simulink model "bbbbbbbb"  (R2018b)
settings: Solver=VariableStepAuto  StartTime=0.0  StopTime=20  MaxStep=0.01  RelTol=1e-3
values from neighbouring files (symbols this model uses):
  A = [0 1; 4 0]    [snatch3.m]    (also in snatch4.m; snatch5.m; snatch6.m)
  B = [1; 1]    [snatch3.m]    (also in snatch4.m; snatch5.m; snatch6.m)
  C = [3 0]    [snatch3.m]    (also in snatch4.m; snatch5.m; snatch6.m)
  D = 3    [snatch3.m]
  K = inv(R)*transpose(B)*P    [snatch3.m]    (also in snatch4.m = [k1Sol(2) k2Sol(2)]; snatch5.m; snatch6.m = [k1Sol(2) k2Sol(2)])
settings Model: Creator=kekos  LastModifiedBy=kekos

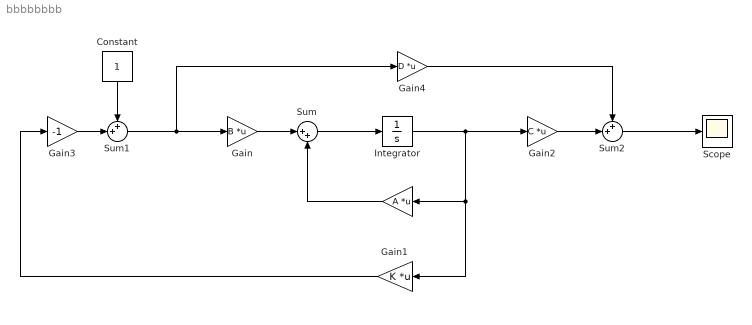
== system bbbbbbbb ==
  " " : Gain  Gain=A  Multiplication=Matrix(K*u)
  Constant : Constant
  Gain : Gain  Gain=B  Multiplication=Matrix(K*u)
  Gain1 : Gain  Gain=K  Multiplication=Matrix(K*u)
  Gain2 : Gain  Gain=C  Multiplication=Matrix(K*u)
  Gain3 : Gain  Gain=-1
  Gain4 : Gain  Gain=D  Multiplication=Matrix(K*u)
  Integrator : Integrator
  Scope : Scope
  Sum : Sum  Inputs=|++
  Sum1 : Sum  Inputs=++|
  Sum2 : Sum  Inputs=++|
  wires:
  Sum1/1 -> Gain4/1, Gain/1
  " "/1 -> Sum/2
  Integrator/1 -> Gain2/1, Gain1/1, " "/1
  Sum/1 -> Integrator/1
  Gain/1 -> Sum/1
  Gain1/1 -> Gain3/1
  Gain3/1 -> Sum1/2
  Gain4/1 -> Sum2/1
  Gain2/1 -> Sum2/2
  Sum2/1 -> Scope/1
  Constant/1 -> Sum1/1
